simulink model "Feeder_1"  (Simulink 8.8)
settings: Solver=ode4  StartTime=0.0  StopTime=inf  FixedStep=Ts  RelTol=1e-3  EnableMultiTasking=on
PreLoadFcn:
  | Ts=125e-6;Core_Num = 0; np=1; nq=1; Vmin=.9;
PostLoadFcn:
  | Ts=125e-6;Core_Num = 0; np=1; nq=1; Vmin=.9;
InitFcn:
  | Ts=125e-6;Core_Num = 0; np=1; nq=1; Vmin=.9;
undefined symbols (not defined in the file or in its folder): another_event_name, DiscIntNeverNeededParam, I, j, Left, my_event_name, Right, type, V, X
libraries: powerlib x316, powerlib_meascontrol x227, simulink_extras x78, simulink x25, rtio_generic_c37_118 x22, ssn_lib x9, rtlab x6, powerlib_extras x3, artemis x1, rtio_opalrt_ml605ex1 x1, rtio_spectracom x1, rtio_generic_ethernet x1
(part 7 of 14)

== system Feeder_1/SM_NG/Subsystem/Single-Phase Voltage Regulator1 ==
  " " : Gain  Gain=-1/ctRatio
  "   " : Terminator
  "    " : Gain  Gain=1/ptRatio
  "        " : powerlib/Elements/Linear Transformer  UNITS=SI  NominalPower=[pNom fNom]  winding1=[vNom/ptRatio 1.152e-007 1.2223e-008]  winding2=[vNom/ptRatio 1.152e-007 1.2223e-008]  ThreeWindings=off  winding3=[3.15e+005 0.7938 0.084225]  RmLm=[1.3824e+005 366.69]  Measurements=None  DataType=on
  "    4" : Gain  Gain=1/sqrt(2)
  Back-Euler : Constant
  CT : powerlib/Measurements/Current Measurement  PhasorSimulation=off  OutputType=Complex  PSBequivalent=0
  "CTS  " : powerlib/Electrical Sources/Controlled Current Source  Initialize=on  Source_Type=AC  Amplitude=0  Phase=0  Frequency=0  Measurements=None
  Constant : Constant  Value=122.4
  Constant1 : Constant  Value=1.25
  Constant2 : Constant  Value=totalDelay
  Constant3 : Constant
  Discrete  Fourier1 : powerlib_extras/Discrete Measurements/Discrete  Fourier  Freq=fNom  n=1  Par_Init=[0 0]  Ts=Ts
  Discrete-Time Integrator : DiscreteIntegrator  SampleTime=-1  ICPrevOutput=DiscIntNeverNeededParam  ICPrevScaledInput=DiscIntNeverNeededParam
  Fcn : Fcn  Expr=1+0.1*u(1)/16
  Ground : powerlib/Elements/Ground  LConnTagsString=a
  Memory : Memory
  Memory1 : Memory
  Mux1 : Mux  Inputs=2
  PT : powerlib/Measurements/Voltage Measurement  PhasorSimulation=off  OutputType=Complex  PSBequivalent=0
  "PTS  " : powerlib/Electrical Sources/Controlled Voltage Source  Initialize=on  Source_Type=AC  Amplitude=0  Phase=0  Frequency=0  Measurements=None
  R+jX : powerlib/Elements/Series RLC Branch  LConnTagsString=__new0  RConnTagsString=__new0  BranchType=RL  Resistance=r  Inductance=x / (2*pi*fNom)  SetiL0=off  InitialCurrent=0  Capacitance=1e-6  Setx0=off  InitialVoltage=0  Measurements=None
  RMS : powerlib_meascontrol/Measurements/RMS  TrueRMS=on  Freq=60  RMSInit=120  Ts=Ts
  Rauxiliary : powerlib/Elements/Series RLC Branch  LConnTagsString=__new0  RConnTagsString=__new0  BranchType=R  Resistance=1e3  Inductance=1.6 / (120*pi)  SetiL0=off  InitialCurrent=0  Capacitance=1e-6  Setx0=off  InitialVoltage=0  Measurements=None
  Regulating logic : MATLAB Function  TreatAsAtomicUnit=on
  SSN Interface Block (1ph) : ssn_lib/SSN Interface Block (1ph)  nb_phase=1  nb_port=2  p1_type=V-type(Left)  p2_type=X-type(Right)  p3_type=V-type(Left)  p4_type=V-type(Left)  p5_type=V-type(Left)  p6_type=V-type(Left)  p7_type=V-type(Left)  p8_type=V-type(Left)  p9_type=V-type(Left)  p10_type=V-type(Left)  p11_type=V-type(Left)  p12_type=V-type(Left)  p13_type=V-type(Left)  p14_type=V-type(Left)  p15_type=V-type(Left)  p16_type=V-type(Left)  I_port_shunt_resistance=1e9
  SSN Interface Block (1ph)2 : ssn_lib/SSN Interface Block (1ph)  nb_phase=1  nb_port=2  p1_type=X-type(Left)  p2_type=I-type(Right)  p3_type=X-type(Left)  p4_type=V-type (Right)  p5_type=V-type(Left)  p6_type=V-type(Left)  p7_type=V-type(Left)  p8_type=V-type(Left)  p9_type=V-type(Left)  p10_type=V-type(Left)  p11_type=V-type(Left)  p12_type=V-type(Left)  p13_type=V-type(Left)  p14_type=V-type(Left)  p15_type=V-type(Left)  p16_type=V-type(Left)  I_port_shunt_resistance=1e9
  SSN OLTC xfo v2 : Subsystem  AncestorBlock=artemis/SSN/SSN OLTC/SSN OLTC xfo v2  mask(Norton-Type External Nodal Subsystem){nnode=2, taggg=58fx9b24xf29057391169, conntype=2 ports, RLpri=[1e-4 1e-5], Rcore=10000, ensat=on, Lcore=1000, Lsat=1000, phisat=1e8, Ts=Ts}
      mask prompts: nnode "Number of Electric nodes"; taggg "Unique Tag Identifier (automatic)"; conntype "Connection type"; RLpri "Primary winding resistance and inductance ([Ohms H])"; Rcore "Core Resistance (Ohms)"; ensat "Enable Saturation"; Lcore "Unsaturated magnetisation inductance (H)"; Lsat "Saturated magnetisation inductance (H)"; phisat "Flux saturation threshold (Weber)"; Ts "Sample Time (s)"
      mask help:
      | Continuously-variable On-Load Tapped Transformer (OLTC) (SSN Custom model)
      |
      | This block implements a 2 winding OLTC saturable transformer in SSN.
      | The model has a variable secondary inductance and resistance as well as turn-ratio.
      | The secondary winding is on the side marked with 'TAP'
      |
      | Mask parameters:
      |    Unique Tag Identifier: unique tag required by SSN to recknonize SSN external models
      |    Primary winding resistance and inductance ([Ohms H])
      |    Core Resistance (Ohms)
      |    Unsaturated magnetisation inductance (H): unsaturated core magnetization inductance
      |    Saturated magnetisation inductance (H): local inductance of the core in the saturated region
      |    Flux saturation threshold (Weber): flux saturation point
      |
      | Signal parameters:
      |
      | Signal inputs:
      |    1st sig: secondary winding resistance (Ohms)
      |    2nd sig: secondary winding inductance (H)
      |    3rd sig: transformer turn ratio k (V_secondary_tapped=k*V_primary)
      |    4th sig:  when set to 1, uses the Backward Euler method for solver. This can be used dynamically during simulation for example to damp numerical oscillations after switching events or after tap changes.
      |
      | Signals ouputs:
      |    1st signal: primary input current (A)
      |    2nd signal: secondary winding current (A)
      |    3rd signal: transformer flux (Wb)
      |
      | Saturation characteristic:
      |          flux
      |             ^              2
      |             |      1       *   <--- slope between point1 and point2 is Lsaturated
      |  phisat  |-----*  <---  this is the knee of flux=f(imag)
      |             |
      |             |
      |             |  <-----slope between origin and point1 is Lunsaturated
      |             *-------------------> imag
      mask init:
      | bloc=gcb;
      | taggg=get_param(bloc,'taggg');
      | conntyp=get_param(bloc,'conntype');
      | set_param([bloc '/FromV'],'GotoTag',['ssn_ext_sys_from_V_' taggg]);
      | set_param([bloc '/GotoHist'],'GotoTag',['ssn_ext_sys_goto_Hist_' taggg]);
      | set_param([bloc '/GotoY'],'GotoTag',['ssn_ext_sys_goto_Y_' taggg]);
      | 
      | R1=RLpri(1);
      | L1=RLpri(2);
      | 
      | if isequal(get_param(bloc,'ensat'),'off')
      |     phisat=1e21;
      | end
      | 
      | if isequal(conntyp,'4 ports')
      |     vin_sel=[1 2 3 4];
      |     Vinzeros=0;
      |     hist_sel=[1 2 3 4];
      |     a1=0;a2=0;a3=100;a4=100; b1=[7,34,40,33,31,33,40,33,31,33,40,33,31,33,40,34,7];b2=[30,30,34,42,40,37,45,52,50,47,54,62,59,57,65,70,70];b3=[93,67,60,67,70,67,60,67,70,67,60,67,70,67,60,67,93];b4=[30,30,34,42,40,37,45,52,50,47,54,62,60,57,65,70,70];
      |     c1=[20,20]*0;c2=[20,30]*0;c3=[27,14]*0;c4=[20,20]*0;c5=[24,17]*0;c6=[16,16]*0;c7=[22,19]*0;c8=[13,13]*0;c9=[80,80]*0;c10=[20,30]*0;c11=[88,74]*0;c12=[20,20]*0;c13=[85,77]*0;c14=[16,16]*0;c15=[81,79]*0;c16=[13,13]*0;
      |     %d1=[85,80];d2=[60,60];d3=[83,83];d4=[50,60];d5=[90,88,86];d6=[50,60,50];d7=[89,87];d8=[54,54];d9=[92,95,96,96,95,92,92];d10=[53,53,55,58,60,60,50];
      | 
      | 
      | elseif isequal(conntyp,'3 ports (primary grounded)')
      |     vin_sel=[1 2 5 3];
      |     Vinzeros=[0 0];
      |     hist_sel=[1 2 4];
      |   
      |      a1=0;a2=0;a3=100;a4=100; b1=[20,34,40,33,31,33,40,33,31,33,40,33,31,33,40,34,7];b2=[30,30,34,42,40,37,45,52,50,47,54,62,59,57,65,70,70];b3=[93,67,60,67,70,67,60,67,70,67,60,67,70,67,60,67,93];b4=[30,30,34,42,40,37,45,52,50,47,54,62,60,57,65,70,70];
      |     c1=[20,20];c2=[20,30];c3=[27,14];c4=[20,20];c5=[24,17];c6=[16,16];c7=[22,19];c8=[13,13];c9=[80,80]*0;c10=[20,30]*0;c11=[88,74]*0;c12=[20,20]*0;c13=[85,77]*0;c14=[16,16]*0;c15=[81,79]*0;c16=[13,13]*0;
      |     %d1=[85,80];d2=[60,60];d3=[83,83];d4=[50,60];d5=[90,88,86];d6=[50,60,50];d7=[89,87];d8=[54,54];d9=[92,95,96,96,95,92,92];d10=[53,53,55,58,60,60,50];
      | elseif isequal(conntyp,'3 ports (tapped secondary grounded)')
      |     vin_sel=[1 2 3 5];
      |     Vinzeros=[0 0];
      |     hist_sel=[1 2 3];
      |  
      |    a1=0;a2=0;a3=100;a4=100; b1=[20,34,40,33,31,33,40,33,31,33,40,33,31,33,40,34,7];b2=[30,30,34,42,40,37,45,52,50,47,54,62,59,57,65,70,70];b3=[80,67,60,67,70,67,60,67,70,67,60,67,70,67,60,67,93];b4=[30,30,34,42,40,37,45,52,50,47,54,62,60,57,65,70,70];
      |     c1=[20,20]*0;c2=[20,30]*0;c3=[27,14]*0;c4=[20,20]*0;c5=[24,17]*0;c6=[16,16]*0;c7=[22,19]*0;c8=[13,13]*0;c9=[80,80];c10=[20,30];c11=[88,74];c12=[20,20];c13=[85,77];c14=[16,16];c15=[81,79];c16=[13,13];
      |     %d1=[85,80];d2=[60,60];d3=[83,83];d4=[50,60];d5=[90,88,86];d6=[50,60,50];d7=[89,87];d8=[54,54];d9=[92,95,96,96,95,92,92];d10=[53,53,55,58,60,60,50];
      | elseif isequal(conntyp,'2 ports')
      |     vin_sel=[1 2 5 5];
      |     Vinzeros=[0 0 0];
      |     hist_sel=[1 2];
      |         a1=0;a2=0;a3=100;a4=100; b1=[20,34,40,33,31,33,40,33,31,33,40,33,31,33,40,34,7];b2=[30,30,34,42,40,37,45,52,50,47,54,62,59,57,65,70,70];b3=[80,67,60,67,70,67,60,67,70,67,60,67,70,67,60,67,93];b4=[30,30,34,42,40,37,45,52,50,47,54,62,60,57,65,70,70];
      |     c1=[20,20];c2=[20,30];c3=[27,14];c4=[20,20];c5=[24,17];c6=[16,16];c7=[22,19];c8=[13,13];c9=[80,80];c10=[20,30];c11=[88,74];c12=[20,20];c13=[85,77];c14=[16,16];c15=[81,79];c16=[13,13];
      |     %d1=[85,80];d2=[60,60];d3=[83,83];d4=[50,60];d5=[90,88,86];d6=[50,60,50];d7=[89,87];d8=[54,54];d9=[92,95,96,96,95,92,92];d10=[53,53,55,58,60,60,50];
      | else
      | 
      | end
      | 
      | ori=get_param(bloc,'Orientation');
      | 
      | if isequal(ori,'right')
      |     d1=[73,67];d2=[56,56];d3=[70,70];d4=[45,56];d5=[80,77,75];d6=[45,56,45];d7=[79,76];d8=[50,50];d9=[82,84,86,84,82,82];d10=[50,50,54,56,56,45];
      | else
      |     d1=[73,71,69,71,73,73];d2=[50,50,52,56,56,45];d3=[80,77,75];d4=[45,56,45];d5=[76,79];d6=[50,50];d7=[88,82];d8=[56,56];d9=[85,85];d10=[45,56];
      | end
      settings: CopyFcn=|
      | str=tempname;
      | str=strrep(str(end-20:end),'_','x');
      | set_param(gcb,'taggg',str);
      | set_param(gcb,'LinkStatus','inactive');
      mask Help: eval('open SSN_OLTC.pdf;');
      mask TypeOptions conntype: 4 ports | 3 ports (primary grounded) | 3 ports (tapped secondary grounded) | 2 ports
      mask Callback conntype:
      | bloc=gcb;
      | conntyp=get_param(bloc,'conntype');
      | nn=fts6_xfo_port_cb(bloc,conntyp);
      | set_param(bloc,'nnode',nn);
      mask Display:
      | plot(a1,a2,a3,a4,b1,b2,b3,b4,c1,c2,c3,c4,c5,c6,c7,c8,c9,c10,c11,c12,c13,c14,c15,c16);
      | color('blue');
      | plot(d1,d2,d3,d4,d5,d6,d7,d8,d9,d10);
  Terminator : Terminator
  Transfo R2-L2-turnratio : Constant  Value=[0.0001 0.00001 1]
  VRelay : powerlib/Measurements/Voltage Measurement  PhasorSimulation=off  OutputType=Complex  PSBequivalent=0
  x : Product  RndMeth=Zero
  Source Side : PMIOPort  Port=1  Side=Left
  Load Side : PMIOPort  Port=2  Side=Right
  tapNo : Outport
  wires:
  CT/1 -> " "/1
  " "/1 -> Memory/1
  PT/1 -> "    "/1
  "    "/1 -> Memory1/1
  [CTS] -> "CTS  "/1
  [PTS] -> RMS/1, "PTS  "/1
  VRelay/1 -> Discrete  Fourier1/1
  Discrete  Fourier1/1 -> "    4"/1
  Discrete-Time Integrator/1 -> Regulating logic/5(clock)
  Regulating logic/1(tapNumberOut) -> [tapNo], tapNo/1
  Constant/1 -> Regulating logic/2(vRef)
  Constant1/1 -> Regulating logic/3(bandwidth)
  Constant2/1 -> Regulating logic/4(delayTime)
  Memory/1 -> [CTS]
  Memory1/1 -> [PTS]
  Discrete  Fourier1/2 -> Terminator/1
  Back-Euler/1 -> Mux1/2
  Transfo R2-L2-turnratio/1 -> x/2
  x/1 -> Mux1/1
  Fcn/1 -> x/1
  [tapNo] -> Fcn/1
  Constant3/1 -> Discrete-Time Integrator/1
  RMS/1 -> Regulating logic/1(vRelay)
  Mux1/1 -> SSN OLTC xfo v2/1(params)
  SSN OLTC xfo v2/1(meas) -> "   "/1
  connections:
  R+jX/LConn1 -- "        "/LConn1 -- "CTS  "/RConn1 -- Rauxiliary/LConn1
  R+jX/RConn1 -- "        "/LConn2 -- "CTS  "/LConn1 -- Rauxiliary/RConn1
  "PTS  "/RConn1 -- "        "/RConn1
  "        "/RConn2 -- VRelay/LConn1
  PT/LConn1 -- CT/RConn1 -- SSN Interface Block (1ph)2/RConn1
  PT/LConn2 -- Ground/LConn1
  VRelay/LConn2 -- "PTS  "/LConn1
  Load Side/RConn1 -- CT/LConn1
  SSN Interface Block (1ph)/RConn1 -- SSN OLTC xfo v2/LConn1
  SSN Interface Block (1ph)2/LConn1 -- SSN OLTC xfo v2/RConn1
  SSN Interface Block (1ph)/LConn1 -- Source Side/RConn1

== system Feeder_1/SM_NG/Subsystem/Single-Phase Voltage Regulator2 ==
  " " : Gain  Gain=-1/ctRatio
  "   " : Terminator
  "    " : Gain  Gain=1/ptRatio
  "        " : powerlib/Elements/Linear Transformer  UNITS=SI  NominalPower=[pNom fNom]  winding1=[vNom/ptRatio 1.152e-007 1.2223e-008]  winding2=[vNom/ptRatio 1.152e-007 1.2223e-008]  ThreeWindings=off  winding3=[3.15e+005 0.7938 0.084225]  RmLm=[1.3824e+005 366.69]  Measurements=None  DataType=on
  "    4" : Gain  Gain=1/sqrt(2)
  Back-Euler : Constant
  CT : powerlib/Measurements/Current Measurement  PhasorSimulation=off  OutputType=Complex  PSBequivalent=0
  "CTS  " : powerlib/Electrical Sources/Controlled Current Source  Initialize=on  Source_Type=AC  Amplitude=0  Phase=0  Frequency=0  Measurements=None
  Constant : Constant  Value=122.4
  Constant1 : Constant  Value=1.25
  Constant2 : Constant  Value=totalDelay
  Constant3 : Constant
  Discrete  Fourier1 : powerlib_extras/Discrete Measurements/Discrete  Fourier  Freq=fNom  n=1  Par_Init=[0 0]  Ts=Ts
  Discrete-Time Integrator : DiscreteIntegrator  SampleTime=-1  ICPrevOutput=DiscIntNeverNeededParam  ICPrevScaledInput=DiscIntNeverNeededParam
  Fcn : Fcn  Expr=1+0.1*u(1)/16
  Ground : powerlib/Elements/Ground  LConnTagsString=a
  Memory : Memory
  Memory1 : Memory
  Mux1 : Mux  Inputs=2
  PT : powerlib/Measurements/Voltage Measurement  PhasorSimulation=off  OutputType=Complex  PSBequivalent=0
  "PTS  " : powerlib/Electrical Sources/Controlled Voltage Source  Initialize=on  Source_Type=AC  Amplitude=0  Phase=0  Frequency=0  Measurements=None
  R+jX : powerlib/Elements/Series RLC Branch  LConnTagsString=__new0  RConnTagsString=__new0  BranchType=RL  Resistance=r  Inductance=x / (2*pi*fNom)  SetiL0=off  InitialCurrent=0  Capacitance=1e-6  Setx0=off  InitialVoltage=0  Measurements=None
  RMS : powerlib_meascontrol/Measurements/RMS  TrueRMS=on  Freq=60  RMSInit=120  Ts=Ts
  Rauxiliary : powerlib/Elements/Series RLC Branch  LConnTagsString=__new0  RConnTagsString=__new0  BranchType=R  Resistance=1e3  Inductance=1.6 / (120*pi)  SetiL0=off  InitialCurrent=0  Capacitance=1e-6  Setx0=off  InitialVoltage=0  Measurements=None
  Regulating logic : MATLAB Function  TreatAsAtomicUnit=on
  SSN Interface Block (1ph) : ssn_lib/SSN Interface Block (1ph)  nb_phase=1  nb_port=2  p1_type=V-type(Left)  p2_type=X-type(Right)  p3_type=V-type(Left)  p4_type=V-type(Left)  p5_type=V-type(Left)  p6_type=V-type(Left)  p7_type=V-type(Left)  p8_type=V-type(Left)  p9_type=V-type(Left)  p10_type=V-type(Left)  p11_type=V-type(Left)  p12_type=V-type(Left)  p13_type=V-type(Left)  p14_type=V-type(Left)  p15_type=V-type(Left)  p16_type=V-type(Left)  I_port_shunt_resistance=1e9
  SSN Interface Block (1ph)2 : ssn_lib/SSN Interface Block (1ph)  nb_phase=1  nb_port=2  p1_type=X-type(Left)  p2_type=I-type(Right)  p3_type=X-type(Left)  p4_type=V-type (Right)  p5_type=V-type(Left)  p6_type=V-type(Left)  p7_type=V-type(Left)  p8_type=V-type(Left)  p9_type=V-type(Left)  p10_type=V-type(Left)  p11_type=V-type(Left)  p12_type=V-type(Left)  p13_type=V-type(Left)  p14_type=V-type(Left)  p15_type=V-type(Left)  p16_type=V-type(Left)  I_port_shunt_resistance=1e9
  SSN OLTC xfo v2 : Subsystem  AncestorBlock=artemis/SSN/SSN OLTC/SSN OLTC xfo v2  mask(Norton-Type External Nodal Subsystem){nnode=2, taggg=081xa09bxd1beaba51875, conntype=2 ports, RLpri=[1e-4 1e-5], Rcore=10000, ensat=on, Lcore=1000, Lsat=1000, phisat=1e8, Ts=Ts}
      mask prompts: nnode "Number of Electric nodes"; taggg "Unique Tag Identifier (automatic)"; conntype "Connection type"; RLpri "Primary winding resistance and inductance ([Ohms H])"; Rcore "Core Resistance (Ohms)"; ensat "Enable Saturation"; Lcore "Unsaturated magnetisation inductance (H)"; Lsat "Saturated magnetisation inductance (H)"; phisat "Flux saturation threshold (Weber)"; Ts "Sample Time (s)"
      mask help:
      | Continuously-variable On-Load Tapped Transformer (OLTC) (SSN Custom model)
      |
      | This block implements a 2 winding OLTC saturable transformer in SSN.
      | The model has a variable secondary inductance and resistance as well as turn-ratio.
      | The secondary winding is on the side marked with 'TAP'
      |
      | Mask parameters:
      |    Unique Tag Identifier: unique tag required by SSN to recknonize SSN external models
      |    Primary winding resistance and inductance ([Ohms H])
      |    Core Resistance (Ohms)
      |    Unsaturated magnetisation inductance (H): unsaturated core magnetization inductance
      |    Saturated magnetisation inductance (H): local inductance of the core in the saturated region
      |    Flux saturation threshold (Weber): flux saturation point
      |
      | Signal parameters:
      |
      | Signal inputs:
      |    1st sig: secondary winding resistance (Ohms)
      |    2nd sig: secondary winding inductance (H)
      |    3rd sig: transformer turn ratio k (V_secondary_tapped=k*V_primary)
      |    4th sig:  when set to 1, uses the Backward Euler method for solver. This can be used dynamically during simulation for example to damp numerical oscillations after switching events or after tap changes.
      |
      | Signals ouputs:
      |    1st signal: primary input current (A)
      |    2nd signal: secondary winding current (A)
      |    3rd signal: transformer flux (Wb)
      |
      | Saturation characteristic:
      |          flux
      |             ^              2
      |             |      1       *   <--- slope between point1 and point2 is Lsaturated
      |  phisat  |-----*  <---  this is the knee of flux=f(imag)
      |             |
      |             |
      |             |  <-----slope between origin and point1 is Lunsaturated
      |             *-------------------> imag
      mask init: same as Feeder_1/SM_NG/Subsystem/Single-Phase Voltage Regulator1/SSN OLTC xfo v2
      settings: CopyFcn=|
      | str=tempname;
      | str=strrep(str(end-20:end),'_','x');
      | set_param(gcb,'taggg',str);
      | set_param(gcb,'LinkStatus','inactive');
      mask Help: eval('open SSN_OLTC.pdf;');
      mask TypeOptions conntype: 4 ports | 3 ports (primary grounded) | 3 ports (tapped secondary grounded) | 2 ports
      mask Callback conntype:
      | bloc=gcb;
      | conntyp=get_param(bloc,'conntype');
      | nn=fts6_xfo_port_cb(bloc,conntyp);
      | set_param(bloc,'nnode',nn);
      mask Display:
      | plot(a1,a2,a3,a4,b1,b2,b3,b4,c1,c2,c3,c4,c5,c6,c7,c8,c9,c10,c11,c12,c13,c14,c15,c16);
      | color('blue');
      | plot(d1,d2,d3,d4,d5,d6,d7,d8,d9,d10);
  Terminator : Terminator
  Transfo R2-L2-turnratio : Constant  Value=[0.0001 0.00001 1]
  VRelay : powerlib/Measurements/Voltage Measurement  PhasorSimulation=off  OutputType=Complex  PSBequivalent=0
  x : Product  RndMeth=Zero
  Source Side : PMIOPort  Port=1  Side=Left
  Load Side : PMIOPort  Port=2  Side=Right
  tapNo : Outport
  wires:
  CT/1 -> " "/1
  " "/1 -> Memory/1
  PT/1 -> "    "/1
  "    "/1 -> Memory1/1
  [CTS] -> "CTS  "/1
  [PTS] -> RMS/1, "PTS  "/1
  VRelay/1 -> Discrete  Fourier1/1
  Discrete  Fourier1/1 -> "    4"/1
  Discrete-Time Integrator/1 -> Regulating logic/5(clock)
  Regulating logic/1(tapNumberOut) -> [tapNo], tapNo/1
  Constant/1 -> Regulating logic/2(vRef)
  Constant1/1 -> Regulating logic/3(bandwidth)
  Constant2/1 -> Regulating logic/4(delayTime)
  Memory/1 -> [CTS]
  Memory1/1 -> [PTS]
  Discrete  Fourier1/2 -> Terminator/1
  Back-Euler/1 -> Mux1/2
  Transfo R2-L2-turnratio/1 -> x/2
  x/1 -> Mux1/1
  Fcn/1 -> x/1
  [tapNo] -> Fcn/1
  Constant3/1 -> Discrete-Time Integrator/1
  RMS/1 -> Regulating logic/1(vRelay)
  Mux1/1 -> SSN OLTC xfo v2/1(params)
  SSN OLTC xfo v2/1(meas) -> "   "/1
  connections:
  R+jX/LConn1 -- "        "/LConn1 -- "CTS  "/RConn1 -- Rauxiliary/LConn1
  R+jX/RConn1 -- "        "/LConn2 -- "CTS  "/LConn1 -- Rauxiliary/RConn1
  "PTS  "/RConn1 -- "        "/RConn1
  "        "/RConn2 -- VRelay/LConn1
  PT/LConn1 -- CT/RConn1 -- SSN Interface Block (1ph)2/RConn1
  PT/LConn2 -- Ground/LConn1
  VRelay/LConn2 -- "PTS  "/LConn1
  Load Side/RConn1 -- CT/LConn1
  SSN Interface Block (1ph)/RConn1 -- SSN OLTC xfo v2/LConn1
  SSN Interface Block (1ph)2/LConn1 -- SSN OLTC xfo v2/RConn1
  SSN Interface Block (1ph)/LConn1 -- Source Side/RConn1

== system Feeder_1/SM_NG/Subsystem/Single-Phase Voltage Regulator3 ==
  " " : Gain  Gain=-1/ctRatio
  "   " : Terminator
  "    " : Gain  Gain=1/ptRatio
  "        " : powerlib/Elements/Linear Transformer  UNITS=SI  NominalPower=[pNom fNom]  winding1=[vNom/ptRatio 1.152e-007 1.2223e-008]  winding2=[vNom/ptRatio 1.152e-007 1.2223e-008]  ThreeWindings=off  winding3=[3.15e+005 0.7938 0.084225]  RmLm=[1.3824e+005 366.69]  Measurements=None  DataType=on
  "    4" : Gain  Gain=1/sqrt(2)
  Back-Euler : Constant
  CT : powerlib/Measurements/Current Measurement  PhasorSimulation=off  OutputType=Complex  PSBequivalent=0
  "CTS  " : powerlib/Electrical Sources/Controlled Current Source  Initialize=on  Source_Type=AC  Amplitude=0  Phase=0  Frequency=0  Measurements=None
  Constant : Constant  Value=122.4
  Constant1 : Constant  Value=1.25
  Constant2 : Constant  Value=totalDelay
  Constant3 : Constant
  Discrete  Fourier1 : powerlib_extras/Discrete Measurements/Discrete  Fourier  Freq=fNom  n=1  Par_Init=[0 0]  Ts=Ts
  Discrete-Time Integrator : DiscreteIntegrator  SampleTime=-1  ICPrevOutput=DiscIntNeverNeededParam  ICPrevScaledInput=DiscIntNeverNeededParam
  Fcn : Fcn  Expr=1+0.1*u(1)/16
  Ground : powerlib/Elements/Ground  LConnTagsString=a
  Memory : Memory
  Memory1 : Memory
  Mux1 : Mux  Inputs=2
  PT : powerlib/Measurements/Voltage Measurement  PhasorSimulation=off  OutputType=Complex  PSBequivalent=0
  "PTS  " : powerlib/Electrical Sources/Controlled Voltage Source  Initialize=on  Source_Type=AC  Amplitude=0  Phase=0  Frequency=0  Measurements=None
  R+jX : powerlib/Elements/Series RLC Branch  LConnTagsString=__new0  RConnTagsString=__new0  BranchType=RL  Resistance=r  Inductance=x / (2*pi*fNom)  SetiL0=off  InitialCurrent=0  Capacitance=1e-6  Setx0=off  InitialVoltage=0  Measurements=None
  RMS : powerlib_meascontrol/Measurements/RMS  TrueRMS=on  Freq=60  RMSInit=120  Ts=Ts
  Rauxiliary : powerlib/Elements/Series RLC Branch  LConnTagsString=__new0  RConnTagsString=__new0  BranchType=R  Resistance=1e3  Inductance=1.6 / (120*pi)  SetiL0=off  InitialCurrent=0  Capacitance=1e-6  Setx0=off  InitialVoltage=0  Measurements=None
  Regulating logic : MATLAB Function  TreatAsAtomicUnit=on
  SSN Interface Block (1ph) : ssn_lib/SSN Interface Block (1ph)  nb_phase=1  nb_port=2  p1_type=V-type(Left)  p2_type=X-type(Right)  p3_type=V-type(Left)  p4_type=V-type(Left)  p5_type=V-type(Left)  p6_type=V-type(Left)  p7_type=V-type(Left)  p8_type=V-type(Left)  p9_type=V-type(Left)  p10_type=V-type(Left)  p11_type=V-type(Left)  p12_type=V-type(Left)  p13_type=V-type(Left)  p14_type=V-type(Left)  p15_type=V-type(Left)  p16_type=V-type(Left)  I_port_shunt_resistance=1e9
  SSN Interface Block (1ph)2 : ssn_lib/SSN Interface Block (1ph)  nb_phase=1  nb_port=2  p1_type=X-type(Left)  p2_type=I-type(Right)  p3_type=X-type(Left)  p4_type=V-type (Right)  p5_type=V-type(Left)  p6_type=V-type(Left)  p7_type=V-type(Left)  p8_type=V-type(Left)  p9_type=V-type(Left)  p10_type=V-type(Left)  p11_type=V-type(Left)  p12_type=V-type(Left)  p13_type=V-type(Left)  p14_type=V-type(Left)  p15_type=V-type(Left)  p16_type=V-type(Left)  I_port_shunt_resistance=1e9
  SSN OLTC xfo v2 : Subsystem  AncestorBlock=artemis/SSN/SSN OLTC/SSN OLTC xfo v2  mask(Norton-Type External Nodal Subsystem){nnode=2, taggg=e32xb02fxc50b2a824a30, conntype=2 ports, RLpri=[1e-4 1e-5], Rcore=10000, ensat=on, Lcore=1000, Lsat=1000, phisat=1e8, Ts=Ts}
      mask prompts: nnode "Number of Electric nodes"; taggg "Unique Tag Identifier (automatic)"; conntype "Connection type"; RLpri "Primary winding resistance and inductance ([Ohms H])"; Rcore "Core Resistance (Ohms)"; ensat "Enable Saturation"; Lcore "Unsaturated magnetisation inductance (H)"; Lsat "Saturated magnetisation inductance (H)"; phisat "Flux saturation threshold (Weber)"; Ts "Sample Time (s)"
      mask help:
      | Continuously-variable On-Load Tapped Transformer (OLTC) (SSN Custom model)
      |
      | This block implements a 2 winding OLTC saturable transformer in SSN.
      | The model has a variable secondary inductance and resistance as well as turn-ratio.
      | The secondary winding is on the side marked with 'TAP'
      |
      | Mask parameters:
      |    Unique Tag Identifier: unique tag required by SSN to recknonize SSN external models
      |    Primary winding resistance and inductance ([Ohms H])
      |    Core Resistance (Ohms)
      |    Unsaturated magnetisation inductance (H): unsaturated core magnetization inductance
      |    Saturated magnetisation inductance (H): local inductance of the core in the saturated region
      |    Flux saturation threshold (Weber): flux saturation point
      |
      | Signal parameters:
      |
      | Signal inputs:
      |    1st sig: secondary winding resistance (Ohms)
      |    2nd sig: secondary winding inductance (H)
      |    3rd sig: transformer turn ratio k (V_secondary_tapped=k*V_primary)
      |    4th sig:  when set to 1, uses the Backward Euler method for solver. This can be used dynamically during simulation for example to damp numerical oscillations after switching events or after tap changes.
      |
      | Signals ouputs:
      |    1st signal: primary input current (A)
      |    2nd signal: secondary winding current (A)
      |    3rd signal: transformer flux (Wb)
      |
      | Saturation characteristic:
      |          flux
      |             ^              2
      |             |      1       *   <--- slope between point1 and point2 is Lsaturated
      |  phisat  |-----*  <---  this is the knee of flux=f(imag)
      |             |
      |             |
      |             |  <-----slope between origin and point1 is Lunsaturated
      |             *-------------------> imag
      mask init: same as Feeder_1/SM_NG/Subsystem/Single-Phase Voltage Regulator1/SSN OLTC xfo v2
      settings: CopyFcn=|
      | str=tempname;
      | str=strrep(str(end-20:end),'_','x');
      | set_param(gcb,'taggg',str);
      | set_param(gcb,'LinkStatus','inactive');
      mask Help: eval('open SSN_OLTC.pdf;');
      mask TypeOptions conntype: 4 ports | 3 ports (primary grounded) | 3 ports (tapped secondary grounded) | 2 ports
      mask Callback conntype:
      | bloc=gcb;
      | conntyp=get_param(bloc,'conntype');
      | nn=fts6_xfo_port_cb(bloc,conntyp);
      | set_param(bloc,'nnode',nn);
      mask Display:
      | plot(a1,a2,a3,a4,b1,b2,b3,b4,c1,c2,c3,c4,c5,c6,c7,c8,c9,c10,c11,c12,c13,c14,c15,c16);
      | color('blue');
      | plot(d1,d2,d3,d4,d5,d6,d7,d8,d9,d10);
  Terminator : Terminator
  Transfo R2-L2-turnratio : Constant  Value=[0.0001 0.00001 1]
  VRelay : powerlib/Measurements/Voltage Measurement  PhasorSimulation=off  OutputType=Complex  PSBequivalent=0
  x : Product  RndMeth=Zero
  Source Side : PMIOPort  Port=1  Side=Left
  Load Side : PMIOPort  Port=2  Side=Right
  tapNo : Outport
  wires:
  CT/1 -> " "/1
  " "/1 -> Memory/1
  PT/1 -> "    "/1
  "    "/1 -> Memory1/1
  [CTS] -> "CTS  "/1
  [PTS] -> RMS/1, "PTS  "/1
  VRelay/1 -> Discrete  Fourier1/1
  Discrete  Fourier1/1 -> "    4"/1
  Discrete-Time Integrator/1 -> Regulating logic/5(clock)
  Regulating logic/1(tapNumberOut) -> [tapNo], tapNo/1
  Constant/1 -> Regulating logic/2(vRef)
  Constant1/1 -> Regulating logic/3(bandwidth)
  Constant2/1 -> Regulating logic/4(delayTime)
  Memory/1 -> [CTS]
  Memory1/1 -> [PTS]
  Discrete  Fourier1/2 -> Terminator/1
  Back-Euler/1 -> Mux1/2
  Transfo R2-L2-turnratio/1 -> x/2
  x/1 -> Mux1/1
  Fcn/1 -> x/1
  [tapNo] -> Fcn/1
  Constant3/1 -> Discrete-Time Integrator/1
  RMS/1 -> Regulating logic/1(vRelay)
  Mux1/1 -> SSN OLTC xfo v2/1(params)
  SSN OLTC xfo v2/1(meas) -> "   "/1
  connections:
  R+jX/LConn1 -- "        "/LConn1 -- "CTS  "/RConn1 -- Rauxiliary/LConn1
  R+jX/RConn1 -- "        "/LConn2 -- "CTS  "/LConn1 -- Rauxiliary/RConn1
  "PTS  "/RConn1 -- "        "/RConn1
  "        "/RConn2 -- VRelay/LConn1
  PT/LConn1 -- CT/RConn1 -- SSN Interface Block (1ph)2/RConn1
  PT/LConn2 -- Ground/LConn1
  VRelay/LConn2 -- "PTS  "/LConn1
  Load Side/RConn1 -- CT/LConn1
  SSN Interface Block (1ph)/RConn1 -- SSN OLTC xfo v2/LConn1
  SSN Interface Block (1ph)2/LConn1 -- SSN OLTC xfo v2/RConn1
  SSN Interface Block (1ph)/LConn1 -- Source Side/RConn1

== system Feeder_1/SS_PMU/Subsystem1/Subsystem ==
  Measurements1 : Inport
  Demux7 : Demux  Outputs=2
  Subsystem1 : Subsystem
  Phasors_Vabc : Outport
  Phasors_Iabc : Outport  Port=2
  Phasor_Freq : Outport  Port=3
  Phasor_DTFreq : Outport  Port=4
  wires:
  Measurements1/1 -> Subsystem1/1(Measurements)
  Subsystem1/2(Phasors_Freq) -> Phasor_Freq/1
  Subsystem1/3(Phasors_DTFreq) -> Phasor_DTFreq/1
  Demux7/2 -> Phasors_Iabc/1
  Demux7/1 -> Phasors_Vabc/1
  Subsystem1/1(Phasors_abc) -> Demux7/1

== system Feeder_1/SS_PMU/Subsystem10/Subsystem ==
  Measurements1 : Inport
  Demux7 : Demux  Outputs=2
  Subsystem1 : Subsystem
  Phasors_Vabc : Outport
  Phasors_Iabc : Outport  Port=2
  Phasor_Freq : Outport  Port=3
  Phasor_DTFreq : Outport  Port=4
  wires:
  Measurements1/1 -> Subsystem1/1(Measurements)
  Subsystem1/2(Phasors_Freq) -> Phasor_Freq/1
  Subsystem1/3(Phasors_DTFreq) -> Phasor_DTFreq/1
  Demux7/2 -> Phasors_Iabc/1
  Demux7/1 -> Phasors_Vabc/1
  Subsystem1/1(Phasors_abc) -> Demux7/1

== system Feeder_1/SS_PMU/Subsystem11/Subsystem ==
  Measurements1 : Inport
  Demux7 : Demux  Outputs=2
  Subsystem1 : Subsystem
  Phasors_Vabc : Outport
  Phasors_Iabc : Outport  Port=2
  Phasor_Freq : Outport  Port=3
  Phasor_DTFreq : Outport  Port=4
  wires:
  Measurements1/1 -> Subsystem1/1(Measurements)
  Subsystem1/2(Phasors_Freq) -> Phasor_Freq/1
  Subsystem1/3(Phasors_DTFreq) -> Phasor_DTFreq/1
  Demux7/2 -> Phasors_Iabc/1
  Demux7/1 -> Phasors_Vabc/1
  Subsystem1/1(Phasors_abc) -> Demux7/1

== system Feeder_1/SS_PMU/Subsystem12/Subsystem ==
  Measurements1 : Inport
  Demux7 : Demux  Outputs=2
  Subsystem1 : Subsystem
  Phasors_Vabc : Outport
  Phasors_Iabc : Outport  Port=2
  Phasor_Freq : Outport  Port=3
  Phasor_DTFreq : Outport  Port=4
  wires:
  Measurements1/1 -> Subsystem1/1(Measurements)
  Subsystem1/2(Phasors_Freq) -> Phasor_Freq/1
  Subsystem1/3(Phasors_DTFreq) -> Phasor_DTFreq/1
  Demux7/2 -> Phasors_Iabc/1
  Demux7/1 -> Phasors_Vabc/1
  Subsystem1/1(Phasors_abc) -> Demux7/1

== system Feeder_1/SS_PMU/Subsystem13/Subsystem ==
  Measurements1 : Inport
  Demux7 : Demux  Outputs=2
  Subsystem1 : Subsystem
  Phasors_Vabc : Outport
  Phasors_Iabc : Outport  Port=2
  Phasor_Freq : Outport  Port=3
  Phasor_DTFreq : Outport  Port=4
  wires:
  Measurements1/1 -> Subsystem1/1(Measurements)
  Subsystem1/2(Phasors_Freq) -> Phasor_Freq/1
  Subsystem1/3(Phasors_DTFreq) -> Phasor_DTFreq/1
  Demux7/2 -> Phasors_Iabc/1
  Demux7/1 -> Phasors_Vabc/1
  Subsystem1/1(Phasors_abc) -> Demux7/1

== system Feeder_1/SS_PMU/Subsystem14/Subsystem ==
  Measurements1 : Inport
  Demux7 : Demux  Outputs=2
  Subsystem1 : Subsystem
  Phasors_Vabc : Outport
  Phasors_Iabc : Outport  Port=2
  Phasor_Freq : Outport  Port=3
  Phasor_DTFreq : Outport  Port=4
  wires:
  Measurements1/1 -> Subsystem1/1(Measurements)
  Subsystem1/2(Phasors_Freq) -> Phasor_Freq/1
  Subsystem1/3(Phasors_DTFreq) -> Phasor_DTFreq/1
  Demux7/2 -> Phasors_Iabc/1
  Demux7/1 -> Phasors_Vabc/1
  Subsystem1/1(Phasors_abc) -> Demux7/1

== system Feeder_1/SS_PMU/Subsystem15/Subsystem ==
  Measurements1 : Inport
  Demux7 : Demux  Outputs=2
  Subsystem1 : Subsystem
  Phasors_Vabc : Outport
  Phasors_Iabc : Outport  Port=2
  Phasor_Freq : Outport  Port=3
  Phasor_DTFreq : Outport  Port=4
  wires:
  Measurements1/1 -> Subsystem1/1(Measurements)
  Subsystem1/2(Phasors_Freq) -> Phasor_Freq/1
  Subsystem1/3(Phasors_DTFreq) -> Phasor_DTFreq/1
  Demux7/2 -> Phasors_Iabc/1
  Demux7/1 -> Phasors_Vabc/1
  Subsystem1/1(Phasors_abc) -> Demux7/1

== system Feeder_1/SS_PMU/Subsystem16/Subsystem ==
  Measurements1 : Inport
  Demux7 : Demux  Outputs=2
  Subsystem1 : Subsystem
  Phasors_Vabc : Outport
  Phasors_Iabc : Outport  Port=2
  Phasor_Freq : Outport  Port=3
  Phasor_DTFreq : Outport  Port=4
  wires:
  Measurements1/1 -> Subsystem1/1(Measurements)
  Subsystem1/2(Phasors_Freq) -> Phasor_Freq/1
  Subsystem1/3(Phasors_DTFreq) -> Phasor_DTFreq/1
  Demux7/2 -> Phasors_Iabc/1
  Demux7/1 -> Phasors_Vabc/1
  Subsystem1/1(Phasors_abc) -> Demux7/1

== system Feeder_1/SS_PMU/Subsystem17/Subsystem ==
  Measurements1 : Inport
  Demux7 : Demux  Outputs=2
  Subsystem1 : Subsystem
  Phasors_Vabc : Outport
  Phasors_Iabc : Outport  Port=2
  Phasor_Freq : Outport  Port=3
  Phasor_DTFreq : Outport  Port=4
  wires:
  Measurements1/1 -> Subsystem1/1(Measurements)
  Subsystem1/2(Phasors_Freq) -> Phasor_Freq/1
  Subsystem1/3(Phasors_DTFreq) -> Phasor_DTFreq/1
  Demux7/2 -> Phasors_Iabc/1
  Demux7/1 -> Phasors_Vabc/1
  Subsystem1/1(Phasors_abc) -> Demux7/1

== system Feeder_1/SS_PMU/Subsystem18/Subsystem ==
  Measurements1 : Inport
  Demux7 : Demux  Outputs=2
  Subsystem1 : Subsystem
  Phasors_Vabc : Outport
  Phasors_Iabc : Outport  Port=2
  Phasor_Freq : Outport  Port=3
  Phasor_DTFreq : Outport  Port=4
  wires:
  Measurements1/1 -> Subsystem1/1(Measurements)
  Subsystem1/2(Phasors_Freq) -> Phasor_Freq/1
  Subsystem1/3(Phasors_DTFreq) -> Phasor_DTFreq/1
  Demux7/2 -> Phasors_Iabc/1
  Demux7/1 -> Phasors_Vabc/1
  Subsystem1/1(Phasors_abc) -> Demux7/1

== system Feeder_1/SS_PMU/Subsystem19/Subsystem ==
  Measurements1 : Inport
  Demux7 : Demux  Outputs=2
  Subsystem1 : Subsystem
  Phasors_Vabc : Outport
  Phasors_Iabc : Outport  Port=2
  Phasor_Freq : Outport  Port=3
  Phasor_DTFreq : Outport  Port=4
  wires:
  Measurements1/1 -> Subsystem1/1(Measurements)
  Subsystem1/2(Phasors_Freq) -> Phasor_Freq/1
  Subsystem1/3(Phasors_DTFreq) -> Phasor_DTFreq/1
  Demux7/2 -> Phasors_Iabc/1
  Demux7/1 -> Phasors_Vabc/1
  Subsystem1/1(Phasors_abc) -> Demux7/1

== system Feeder_1/SS_PMU/Subsystem2/Subsystem ==
  Measurements1 : Inport
  Demux7 : Demux  Outputs=2
  Subsystem1 : Subsystem
  Phasors_Vabc : Outport
  Phasors_Iabc : Outport  Port=2
  Phasor_Freq : Outport  Port=3
  Phasor_DTFreq : Outport  Port=4
  wires:
  Measurements1/1 -> Subsystem1/1(Measurements)
  Subsystem1/2(Phasors_Freq) -> Phasor_Freq/1
  Subsystem1/3(Phasors_DTFreq) -> Phasor_DTFreq/1
  Demux7/2 -> Phasors_Iabc/1
  Demux7/1 -> Phasors_Vabc/1
  Subsystem1/1(Phasors_abc) -> Demux7/1

== system Feeder_1/SS_PMU/Subsystem20/Subsystem ==
  Measurements1 : Inport
  Demux7 : Demux  Outputs=2
  Subsystem1 : Subsystem
  Phasors_Vabc : Outport
  Phasors_Iabc : Outport  Port=2
  Phasor_Freq : Outport  Port=3
  Phasor_DTFreq : Outport  Port=4
  wires:
  Measurements1/1 -> Subsystem1/1(Measurements)
  Subsystem1/2(Phasors_Freq) -> Phasor_Freq/1
  Subsystem1/3(Phasors_DTFreq) -> Phasor_DTFreq/1
  Demux7/2 -> Phasors_Iabc/1
  Demux7/1 -> Phasors_Vabc/1
  Subsystem1/1(Phasors_abc) -> Demux7/1

== system Feeder_1/SS_PMU/Subsystem21/Subsystem ==
  Measurements1 : Inport
  Demux7 : Demux  Outputs=2
  Subsystem1 : Subsystem
  Phasors_Vabc : Outport
  Phasors_Iabc : Outport  Port=2
  Phasor_Freq : Outport  Port=3
  Phasor_DTFreq : Outport  Port=4
  wires:
  Measurements1/1 -> Subsystem1/1(Measurements)
  Subsystem1/2(Phasors_Freq) -> Phasor_Freq/1
  Subsystem1/3(Phasors_DTFreq) -> Phasor_DTFreq/1
  Demux7/2 -> Phasors_Iabc/1
  Demux7/1 -> Phasors_Vabc/1
  Subsystem1/1(Phasors_abc) -> Demux7/1

== system Feeder_1/SS_PMU/Subsystem22/Subsystem ==
  Measurements1 : Inport
  Demux7 : Demux  Outputs=2
  Subsystem1 : Subsystem
  Phasors_Vabc : Outport
  Phasors_Iabc : Outport  Port=2
  Phasor_Freq : Outport  Port=3
  Phasor_DTFreq : Outport  Port=4
  wires:
  Measurements1/1 -> Subsystem1/1(Measurements)
  Subsystem1/2(Phasors_Freq) -> Phasor_Freq/1
  Subsystem1/3(Phasors_DTFreq) -> Phasor_DTFreq/1
  Demux7/2 -> Phasors_Iabc/1
  Demux7/1 -> Phasors_Vabc/1
  Subsystem1/1(Phasors_abc) -> Demux7/1

== system Feeder_1/SS_PMU/Subsystem23/Subsystem ==
  In1 : Inport
  Bus Creator : BusCreator  Inputs=3
  Selector1 : Selector  InputPortWidth=14  IndexOptions=Index vector (dialog)  Indices=[13]  OutputSizes=1
  Selector2 : Selector  InputPortWidth=14  IndexOptions=Index vector (dialog)  Indices=[14]  OutputSizes=1
  Selector5 : Selector  InputPortWidth=14  IndexOptions=Index vector (dialog)  Indices=[1 2 3 4 5 6 7 8 9 10 11 12]  OutputSizes=1
  Out1 : Outport
  wires:
  In1/1 -> Selector5/1, Selector2/1, Selector1/1
  Selector5/1 -> Bus Creator/1  "Measurements"
  Bus Creator/1 -> Out1/1
  Selector1/1 -> Bus Creator/2  "FREQ"
  Selector2/1 -> Bus Creator/3  "FROC"

== system Feeder_1/SS_PMU/Subsystem24/Subsystem ==
  In1 : Inport
  Bus Creator : BusCreator  Inputs=3
  Selector1 : Selector  InputPortWidth=14  IndexOptions=Index vector (dialog)  Indices=[13]  OutputSizes=1
  Selector2 : Selector  InputPortWidth=14  IndexOptions=Index vector (dialog)  Indices=[14]  OutputSizes=1
  Selector5 : Selector  InputPortWidth=14  IndexOptions=Index vector (dialog)  Indices=[1 2 3 4 5 6 7 8 9 10 11 12]  OutputSizes=1
  Out1 : Outport
  wires:
  In1/1 -> Selector5/1, Selector2/1, Selector1/1
  Selector5/1 -> Bus Creator/1  "Measurements"
  Bus Creator/1 -> Out1/1
  Selector1/1 -> Bus Creator/2  "FREQ"
  Selector2/1 -> Bus Creator/3  "FROC"

== system Feeder_1/SS_PMU/Subsystem25/Subsystem ==
  In1 : Inport
  Bus Creator : BusCreator  Inputs=3
  Selector1 : Selector  InputPortWidth=14  IndexOptions=Index vector (dialog)  Indices=[13]  OutputSizes=1
  Selector2 : Selector  InputPortWidth=14  IndexOptions=Index vector (dialog)  Indices=[14]  OutputSizes=1
  Selector5 : Selector  InputPortWidth=14  IndexOptions=Index vector (dialog)  Indices=[1 2 3 4 5 6 7 8 9 10 11 12]  OutputSizes=1
  Out1 : Outport
  wires:
  In1/1 -> Selector5/1, Selector2/1, Selector1/1
  Selector5/1 -> Bus Creator/1  "Measurements"
  Bus Creator/1 -> Out1/1
  Selector1/1 -> Bus Creator/2  "FREQ"
  Selector2/1 -> Bus Creator/3  "FROC"

== system Feeder_1/SS_PMU/Subsystem26/Subsystem ==
  In1 : Inport
  Bus Creator : BusCreator  Inputs=3
  Selector1 : Selector  InputPortWidth=14  IndexOptions=Index vector (dialog)  Indices=[13]  OutputSizes=1
  Selector2 : Selector  InputPortWidth=14  IndexOptions=Index vector (dialog)  Indices=[14]  OutputSizes=1
  Selector5 : Selector  InputPortWidth=14  IndexOptions=Index vector (dialog)  Indices=[1 2 3 4 5 6 7 8 9 10 11 12]  OutputSizes=1
  Out1 : Outport
  wires:
  In1/1 -> Selector5/1, Selector2/1, Selector1/1
  Selector5/1 -> Bus Creator/1  "Measurements"
  Bus Creator/1 -> Out1/1
  Selector1/1 -> Bus Creator/2  "FREQ"
  Selector2/1 -> Bus Creator/3  "FROC"

== system Feeder_1/SS_PMU/Subsystem27/Subsystem ==
  In1 : Inport
  Bus Creator : BusCreator  Inputs=3
  Selector1 : Selector  InputPortWidth=14  IndexOptions=Index vector (dialog)  Indices=[13]  OutputSizes=1
  Selector2 : Selector  InputPortWidth=14  IndexOptions=Index vector (dialog)  Indices=[14]  OutputSizes=1
  Selector5 : Selector  InputPortWidth=14  IndexOptions=Index vector (dialog)  Indices=[1 2 3 4 5 6 7 8 9 10 11 12]  OutputSizes=1
  Out1 : Outport
  wires:
  In1/1 -> Selector5/1, Selector2/1, Selector1/1
  Selector5/1 -> Bus Creator/1  "Measurements"
  Bus Creator/1 -> Out1/1
  Selector1/1 -> Bus Creator/2  "FREQ"
  Selector2/1 -> Bus Creator/3  "FROC"

== system Feeder_1/SS_PMU/Subsystem28/Subsystem ==
  In1 : Inport
  Bus Creator : BusCreator  Inputs=3
  Selector1 : Selector  InputPortWidth=14  IndexOptions=Index vector (dialog)  Indices=[13]  OutputSizes=1
  Selector2 : Selector  InputPortWidth=14  IndexOptions=Index vector (dialog)  Indices=[14]  OutputSizes=1
  Selector5 : Selector  InputPortWidth=14  IndexOptions=Index vector (dialog)  Indices=[1 2 3 4 5 6 7 8 9 10 11 12]  OutputSizes=1
  Out1 : Outport
  wires:
  In1/1 -> Selector5/1, Selector2/1, Selector1/1
  Selector5/1 -> Bus Creator/1  "Measurements"
  Bus Creator/1 -> Out1/1
  Selector1/1 -> Bus Creator/2  "FREQ"
  Selector2/1 -> Bus Creator/3  "FROC"

== system Feeder_1/SS_PMU/Subsystem29/Subsystem ==
  In1 : Inport
  Bus Creator : BusCreator  Inputs=3
  Selector1 : Selector  InputPortWidth=14  IndexOptions=Index vector (dialog)  Indices=[13]  OutputSizes=1
  Selector2 : Selector  InputPortWidth=14  IndexOptions=Index vector (dialog)  Indices=[14]  OutputSizes=1
  Selector5 : Selector  InputPortWidth=14  IndexOptions=Index vector (dialog)  Indices=[1 2 3 4 5 6 7 8 9 10 11 12]  OutputSizes=1
  Out1 : Outport
  wires:
  In1/1 -> Selector5/1, Selector2/1, Selector1/1
  Selector5/1 -> Bus Creator/1  "Measurements"
  Bus Creator/1 -> Out1/1
  Selector1/1 -> Bus Creator/2  "FREQ"
  Selector2/1 -> Bus Creator/3  "FROC"

== system Feeder_1/SS_PMU/Subsystem3/Subsystem ==
  Measurements1 : Inport
  Demux7 : Demux  Outputs=2
  Subsystem1 : Subsystem
  Phasors_Vabc : Outport
  Phasors_Iabc : Outport  Port=2
  Phasor_Freq : Outport  Port=3
  Phasor_DTFreq : Outport  Port=4
  wires:
  Measurements1/1 -> Subsystem1/1(Measurements)
  Subsystem1/2(Phasors_Freq) -> Phasor_Freq/1
  Subsystem1/3(Phasors_DTFreq) -> Phasor_DTFreq/1
  Demux7/2 -> Phasors_Iabc/1
  Demux7/1 -> Phasors_Vabc/1
  Subsystem1/1(Phasors_abc) -> Demux7/1

== system Feeder_1/SS_PMU/Subsystem30/Subsystem ==
  In1 : Inport
  Bus Creator : BusCreator  Inputs=3
  Selector1 : Selector  InputPortWidth=14  IndexOptions=Index vector (dialog)  Indices=[13]  OutputSizes=1
  Selector2 : Selector  InputPortWidth=14  IndexOptions=Index vector (dialog)  Indices=[14]  OutputSizes=1
  Selector5 : Selector  InputPortWidth=14  IndexOptions=Index vector (dialog)  Indices=[1 2 3 4 5 6 7 8 9 10 11 12]  OutputSizes=1
  Out1 : Outport
  wires:
  In1/1 -> Selector5/1, Selector2/1, Selector1/1
  Selector5/1 -> Bus Creator/1  "Measurements"
  Bus Creator/1 -> Out1/1
  Selector1/1 -> Bus Creator/2  "FREQ"
  Selector2/1 -> Bus Creator/3  "FROC"

== system Feeder_1/SS_PMU/Subsystem31/Subsystem ==
  In1 : Inport
  Bus Creator : BusCreator  Inputs=3
  Selector1 : Selector  InputPortWidth=14  IndexOptions=Index vector (dialog)  Indices=[13]  OutputSizes=1
  Selector2 : Selector  InputPortWidth=14  IndexOptions=Index vector (dialog)  Indices=[14]  OutputSizes=1
  Selector5 : Selector  InputPortWidth=14  IndexOptions=Index vector (dialog)  Indices=[1 2 3 4 5 6 7 8 9 10 11 12]  OutputSizes=1
  Out1 : Outport
  wires:
  In1/1 -> Selector5/1, Selector2/1, Selector1/1
  Selector5/1 -> Bus Creator/1  "Measurements"
  Bus Creator/1 -> Out1/1
  Selector1/1 -> Bus Creator/2  "FREQ"
  Selector2/1 -> Bus Creator/3  "FROC"

== system Feeder_1/SS_PMU/Subsystem32/Subsystem ==
  In1 : Inport
  Bus Creator : BusCreator  Inputs=3
  Selector1 : Selector  InputPortWidth=14  IndexOptions=Index vector (dialog)  Indices=[13]  OutputSizes=1
  Selector2 : Selector  InputPortWidth=14  IndexOptions=Index vector (dialog)  Indices=[14]  OutputSizes=1
  Selector5 : Selector  InputPortWidth=14  IndexOptions=Index vector (dialog)  Indices=[1 2 3 4 5 6 7 8 9 10 11 12]  OutputSizes=1
  Out1 : Outport
  wires:
  In1/1 -> Selector5/1, Selector2/1, Selector1/1
  Selector5/1 -> Bus Creator/1  "Measurements"
  Bus Creator/1 -> Out1/1
  Selector1/1 -> Bus Creator/2  "FREQ"
  Selector2/1 -> Bus Creator/3  "FROC"

== system Feeder_1/SS_PMU/Subsystem33/Subsystem ==
  In1 : Inport
  Bus Creator : BusCreator  Inputs=3
  Selector1 : Selector  InputPortWidth=14  IndexOptions=Index vector (dialog)  Indices=[13]  OutputSizes=1
  Selector2 : Selector  InputPortWidth=14  IndexOptions=Index vector (dialog)  Indices=[14]  OutputSizes=1
  Selector5 : Selector  InputPortWidth=14  IndexOptions=Index vector (dialog)  Indices=[1 2 3 4 5 6 7 8 9 10 11 12]  OutputSizes=1
  Out1 : Outport
  wires:
  In1/1 -> Selector5/1, Selector2/1, Selector1/1
  Selector5/1 -> Bus Creator/1  "Measurements"
  Bus Creator/1 -> Out1/1
  Selector1/1 -> Bus Creator/2  "FREQ"
  Selector2/1 -> Bus Creator/3  "FROC"

== system Feeder_1/SS_PMU/Subsystem34/Subsystem ==
  In1 : Inport
  Bus Creator : BusCreator  Inputs=3
  Selector1 : Selector  InputPortWidth=14  IndexOptions=Index vector (dialog)  Indices=[13]  OutputSizes=1
  Selector2 : Selector  InputPortWidth=14  IndexOptions=Index vector (dialog)  Indices=[14]  OutputSizes=1
  Selector5 : Selector  InputPortWidth=14  IndexOptions=Index vector (dialog)  Indices=[1 2 3 4 5 6 7 8 9 10 11 12]  OutputSizes=1
  Out1 : Outport
  wires:
  In1/1 -> Selector5/1, Selector2/1, Selector1/1
  Selector5/1 -> Bus Creator/1  "Measurements"
  Bus Creator/1 -> Out1/1
  Selector1/1 -> Bus Creator/2  "FREQ"
  Selector2/1 -> Bus Creator/3  "FROC"

== system Feeder_1/SS_PMU/Subsystem35/Subsystem ==
  In1 : Inport
  Bus Creator : BusCreator  Inputs=3
  Selector1 : Selector  InputPortWidth=14  IndexOptions=Index vector (dialog)  Indices=[13]  OutputSizes=1
  Selector2 : Selector  InputPortWidth=14  IndexOptions=Index vector (dialog)  Indices=[14]  OutputSizes=1
  Selector5 : Selector  InputPortWidth=14  IndexOptions=Index vector (dialog)  Indices=[1 2 3 4 5 6 7 8 9 10 11 12]  OutputSizes=1
  Out1 : Outport
  wires:
  In1/1 -> Selector5/1, Selector2/1, Selector1/1
  Selector5/1 -> Bus Creator/1  "Measurements"
  Bus Creator/1 -> Out1/1
  Selector1/1 -> Bus Creator/2  "FREQ"
  Selector2/1 -> Bus Creator/3  "FROC"

== system Feeder_1/SS_PMU/Subsystem36/Subsystem ==
  In1 : Inport
  Bus Creator : BusCreator  Inputs=3
  Selector1 : Selector  InputPortWidth=14  IndexOptions=Index vector (dialog)  Indices=[13]  OutputSizes=1
  Selector2 : Selector  InputPortWidth=14  IndexOptions=Index vector (dialog)  Indices=[14]  OutputSizes=1
  Selector5 : Selector  InputPortWidth=14  IndexOptions=Index vector (dialog)  Indices=[1 2 3 4 5 6 7 8 9 10 11 12]  OutputSizes=1
  Out1 : Outport
  wires:
  In1/1 -> Selector5/1, Selector2/1, Selector1/1
  Selector5/1 -> Bus Creator/1  "Measurements"
  Bus Creator/1 -> Out1/1
  Selector1/1 -> Bus Creator/2  "FREQ"
  Selector2/1 -> Bus Creator/3  "FROC"

== system Feeder_1/SS_PMU/Subsystem37/Subsystem ==
  In1 : Inport
  Bus Creator : BusCreator  Inputs=3
  Selector1 : Selector  InputPortWidth=14  IndexOptions=Index vector (dialog)  Indices=[13]  OutputSizes=1
  Selector2 : Selector  InputPortWidth=14  IndexOptions=Index vector (dialog)  Indices=[14]  OutputSizes=1
  Selector5 : Selector  InputPortWidth=14  IndexOptions=Index vector (dialog)  Indices=[1 2 3 4 5 6 7 8 9 10 11 12]  OutputSizes=1
  Out1 : Outport
  wires:
  In1/1 -> Selector5/1, Selector2/1, Selector1/1
  Selector5/1 -> Bus Creator/1  "Measurements"
  Bus Creator/1 -> Out1/1
  Selector1/1 -> Bus Creator/2  "FREQ"
  Selector2/1 -> Bus Creator/3  "FROC"

== system Feeder_1/SS_PMU/Subsystem38/Subsystem ==
  In1 : Inport
  Bus Creator : BusCreator  Inputs=3
  Selector1 : Selector  InputPortWidth=14  IndexOptions=Index vector (dialog)  Indices=[13]  OutputSizes=1
  Selector2 : Selector  InputPortWidth=14  IndexOptions=Index vector (dialog)  Indices=[14]  OutputSizes=1
  Selector5 : Selector  InputPortWidth=14  IndexOptions=Index vector (dialog)  Indices=[1 2 3 4 5 6 7 8 9 10 11 12]  OutputSizes=1
  Out1 : Outport
  wires:
  In1/1 -> Selector5/1, Selector2/1, Selector1/1
  Selector5/1 -> Bus Creator/1  "Measurements"
  Bus Creator/1 -> Out1/1
  Selector1/1 -> Bus Creator/2  "FREQ"
  Selector2/1 -> Bus Creator/3  "FROC"

== system Feeder_1/SS_PMU/Subsystem39/Subsystem ==
  In1 : Inport
  Bus Creator : BusCreator  Inputs=3
  Selector1 : Selector  InputPortWidth=14  IndexOptions=Index vector (dialog)  Indices=[13]  OutputSizes=1
  Selector2 : Selector  InputPortWidth=14  IndexOptions=Index vector (dialog)  Indices=[14]  OutputSizes=1
  Selector5 : Selector  InputPortWidth=14  IndexOptions=Index vector (dialog)  Indices=[1 2 3 4 5 6 7 8 9 10 11 12]  OutputSizes=1
  Out1 : Outport
  wires:
  In1/1 -> Selector5/1, Selector2/1, Selector1/1
  Selector5/1 -> Bus Creator/1  "Measurements"
  Bus Creator/1 -> Out1/1
  Selector1/1 -> Bus Creator/2  "FREQ"
  Selector2/1 -> Bus Creator/3  "FROC"

== system Feeder_1/SS_PMU/Subsystem4/Subsystem ==
  Measurements1 : Inport
  Demux7 : Demux  Outputs=2
  Subsystem1 : Subsystem
  Phasors_Vabc : Outport
  Phasors_Iabc : Outport  Port=2
  Phasor_Freq : Outport  Port=3
  Phasor_DTFreq : Outport  Port=4
  wires:
  Measurements1/1 -> Subsystem1/1(Measurements)
  Subsystem1/2(Phasors_Freq) -> Phasor_Freq/1
  Subsystem1/3(Phasors_DTFreq) -> Phasor_DTFreq/1
  Demux7/2 -> Phasors_Iabc/1
  Demux7/1 -> Phasors_Vabc/1
  Subsystem1/1(Phasors_abc) -> Demux7/1

== system Feeder_1/SS_PMU/Subsystem40/Subsystem ==
  In1 : Inport
  Bus Creator : BusCreator  Inputs=3
  Selector1 : Selector  InputPortWidth=14  IndexOptions=Index vector (dialog)  Indices=[13]  OutputSizes=1
  Selector2 : Selector  InputPortWidth=14  IndexOptions=Index vector (dialog)  Indices=[14]  OutputSizes=1
  Selector5 : Selector  InputPortWidth=14  IndexOptions=Index vector (dialog)  Indices=[1 2 3 4 5 6 7 8 9 10 11 12]  OutputSizes=1
  Out1 : Outport
  wires:
  In1/1 -> Selector5/1, Selector2/1, Selector1/1
  Selector5/1 -> Bus Creator/1  "Measurements"
  Bus Creator/1 -> Out1/1
  Selector1/1 -> Bus Creator/2  "FREQ"
  Selector2/1 -> Bus Creator/3  "FROC"

== system Feeder_1/SS_PMU/Subsystem41/Subsystem ==
  In1 : Inport
  Bus Creator : BusCreator  Inputs=3
  Selector1 : Selector  InputPortWidth=14  IndexOptions=Index vector (dialog)  Indices=[13]  OutputSizes=1
  Selector2 : Selector  InputPortWidth=14  IndexOptions=Index vector (dialog)  Indices=[14]  OutputSizes=1
  Selector5 : Selector  InputPortWidth=14  IndexOptions=Index vector (dialog)  Indices=[1 2 3 4 5 6 7 8 9 10 11 12]  OutputSizes=1
  Out1 : Outport
  wires:
  In1/1 -> Selector5/1, Selector2/1, Selector1/1
  Selector5/1 -> Bus Creator/1  "Measurements"
  Bus Creator/1 -> Out1/1
  Selector1/1 -> Bus Creator/2  "FREQ"
  Selector2/1 -> Bus Creator/3  "FROC"
